simulink model "BLDC_G431"  (R2021a)
settings: Solver=FixedStepDiscrete  StartTime=0.0  StopTime=6  FixedStep=1e-6  RelTol=1e-3
values from neighbouring files (symbols this model uses):
  fpwm = 10000    [BLDC_G431_M.m]
  G1 = -4000    [BLDC_G431_M.m]
  G2 = 14000    [BLDC_G431_M.m]
  Ki = 450    [BLDC_G431_M.m]
  Kp = 0.45    [BLDC_G431_M.m]
  LBG_K1 = -4000    [BLDC_G431_M.m]
  LBG_K2 = 14000    [BLDC_G431_M.m]
  lbg_pll_w = 50    [BLDC_G431_M.m]
  lbg_speedfilter = 0.3    [BLDC_G431_M.m]
  Ld = 0.8e-3/2    (= 0.0004)    [BLDC_G431_M.m]
  Lq = 0.8e-3/2    (= 0.0004)    [BLDC_G431_M.m]
  OPL_Speed = 1200    [BLDC_G431_M.m]
  OPL_Time = 2    [BLDC_G431_M.m]
  OPL_Torque = 3    [BLDC_G431_M.m]
  Pn = 2    [BLDC_G431_M.m]
  Rs = 0.2    [BLDC_G431_M.m]
  Speed_Ki = 0.0633    [BLDC_G431_M.m]
  Speed_Kp = 0.00867    [BLDC_G431_M.m]
  Speed_PI_OutputMax = 6    [BLDC_G431_M.m]
  Speed_PI_OutputMin = -6    [BLDC_G431_M.m]
  Tpwm = 1/fpwm    (= 0.0001)    [BLDC_G431_M.m]
  UDC = 24    [BLDC_G431_M.m]
undefined symbols (not defined in the file or in its folder): Cosine_table, DiscIntNeverNeededParam, R, Sine_table, SMO_PLL_W
libraries: pid_lib x3, simulink x3, mcbplantlib x1, autolibpmsminterior x1
settings Model: DataDictionary=BLDC57.sldd  Creator=zager  LastModifiedBy=zager
settings OptimizationCC: DefaultParameterBehavior=Inlined  UseDivisionForNetSlopeComputation=on  GainParamInheritBuiltInType=on  UseFloatMulNetSlope=on  InlineInvariantSignals=on  PassReuseOutputArgsAs=Individual arguments  ZeroExternalMemoryAtStartup=off  ZeroInternalMemoryAtStartup=off  NoFixptDivByZeroProtection=on  EfficientFloat2IntCast=on  LifeSpan=1  OptimizeBlockOrder=speed  DifferentSizesBufferReuse=on  EfficientTunableParamExpr=on
settings DebuggingCC: ParameterTunabilityLossMsg=error
settings HardwareCC: ProdBitPerPointer=32  ProdBitPerSizeT=32  ProdBitPerPtrDiffT=32  ProdLargestAtomicInteger=Long  ProdLargestAtomicFloat=Double  ProdWordSize=32  ProdLongLongMode=on  ProdHWDeviceType=NXP->Cortex-M4
settings SFSimCC: MATLABDynamicMemAlloc=off
settings RTWCC: SystemTargetFile=ert.tlc  GenCodeOnly=on  TemplateMakefile=ert_default_tmf  GenerateReport=on  LaunchReport=on
settings CodeAppCC: ForceParamTrailComments=on  IgnoreCustomStorageClasses=off  OperatorAnnotations=on  SimulinkDataObjDesc=on  SFDataObjDesc=on  CustomSymbolStrGlobalVar=rt$N$M  CustomSymbolStrType=$N$M  CustomSymbolStrFcn=$N$M$F  CustomSymbolStrMacro=$N$M  InsertBlockDesc=on
settings ERTTargetCC: TargetLangStandard=C99 (ISO)  IncludeMdlTerminateFcn=off  CombineSignalStateStructs=on  SupportComplex=off  SupportNonInlinedSFcns=on  InlinedParameterPlacement=NonHierarchical  ERTCustomFileTemplate=example_file_process.tlc  ERTFilePackagingFormat=CompactWithDataFile

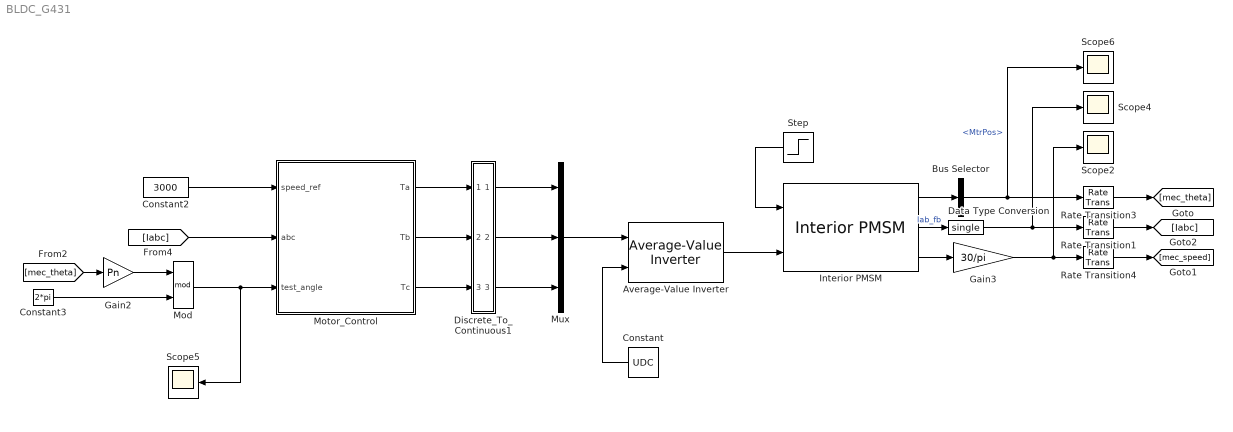
== system BLDC_G431 ==
  Average-Value Inverter : mcbplantlib/Average-Value Inverter
  Bus Selector : BusSelector  OutputSignals=MtrPos
  Constant : Constant  Value=UDC
  Constant2 : Constant  Value=3000  OutDataTypeStr=single
  Constant3 : Constant  Value=2*pi  OutDataTypeStr=single
  Data Type Conversion : DataTypeConversion  OutDataTypeStr=single
  Discrete_To_Continuous1 : Subsystem  Description=""
      mask Display: fprintf('D/C')
  Gain2 : Gain  Gain=Pn  OutDataTypeStr=single
  Gain3 : Gain  Gain=30/pi
  Interior PMSM : autolibpmsminterior/Interior PMSM  port_config=Torque  sim_type=Discrete  Ts=1e-6  P=2  Rs=0.2  Ldq=[0.4e-3 0.4e-3]  KConstText=Back-emf constant (Ke):  lambda_pm=Fluxs  Ke=6.6*sqrt(2)  mechanical=[0.5e-4,8e-5,0]  idq0=[0 0]  theta_init=0  omega_init=0  KConst=6.6*sqrt(2)  lambda_pm_calc=0.02573  Kt=0.07  RefBlkName='autolibpmsminterior/Interior PMSM'  aMode=5
      settings: SourceProductBaseCode=PW,DR,MT,UV,VE
  Mod : Math  Operator=mod  SaturateOnIntegerOverflow=on
  Motor_Control : Subsystem
  Mux : Mux  Inputs=3
  Rate Transition1 : RateTransition  OutPortSampleTime=Tpwm
  Rate Transition3 : RateTransition  OutPortSampleTime=Tpwm
  Rate Transition4 : RateTransition  OutPortSampleTime=Tpwm
  Scope{2,4..6} (4 alike) : Scope
  Step : Step  Time=3  Before=0.1  After=0  SampleTime=0
  wires:
  Constant/1 -> Average-Value Inverter/2
  Average-Value Inverter/1 -> Interior PMSM/2
  Mux/1 -> Average-Value Inverter/1
  Interior PMSM/1 -> Bus Selector/1
  Bus Selector/1 -> Rate Transition3/1, Scope6/1  "<MtrPos>"
  Data Type Conversion/1 -> Rate Transition1/1, Scope4/1
  Interior PMSM/2 -> Data Type Conversion/1  "Iab_fb"
  Discrete_To_Continuous1/1(T1) -> Mux/1
  Discrete_To_Continuous1/2(T2) -> Mux/2
  Discrete_To_Continuous1/3(T3) -> Mux/3
  Rate Transition1/1 -> [Iabc]
  Rate Transition3/1 -> [mec_theta]
  Step/1 -> Interior PMSM/1
  Constant2/1 -> Motor_Control/1(speed_ref)
  [Iabc] -> Motor_Control/2(abc)
  Motor_Control/1(Ta) -> Discrete_To_Continuous1/1(Ta)
  Motor_Control/2(Tb) -> Discrete_To_Continuous1/2(Tb)
  Motor_Control/3(Tc) -> Discrete_To_Continuous1/3(Tc)
  [mec_theta] -> Gain2/1
  Gain2/1 -> Mod/1
  Mod/1 -> Scope5/1, Motor_Control/3(test_angle)
  Rate Transition4/1 -> [mec_speed]
  Interior PMSM/3 -> Gain3/1
  Gain3/1 -> Rate Transition4/1, Scope2/1
  Constant3/1 -> Mod/2

== system BLDC_G431/Discrete_To_Continuous1 ==
  note: Discrete To Continuous
  Ta : Inport
  Tb : Inport  Port=2
  Tc : Inport  Port=3
  DT : DataTypeConversion
  DT1 : DataTypeConversion
  DT2 : DataTypeConversion
  RT : RateTransition  Integrity=off
  RT1 : RateTransition  Integrity=off
  RT2 : RateTransition  Integrity=off
  T1 : Outport
  T2 : Outport  Port=2
  T3 : Outport  Port=3
  wires:
  DT/1 -> RT/1
  Ta/1 -> DT/1  "Tabc"
  DT1/1 -> RT1/1
  Tb/1 -> DT1/1  "Tabc"
  DT2/1 -> RT2/1
  Tc/1 -> DT2/1  "Tabc"
  RT/1 -> T1/1  "Tabc"
  RT1/1 -> T2/1  "Tabc"
  RT2/1 -> T3/1  "Tabc"

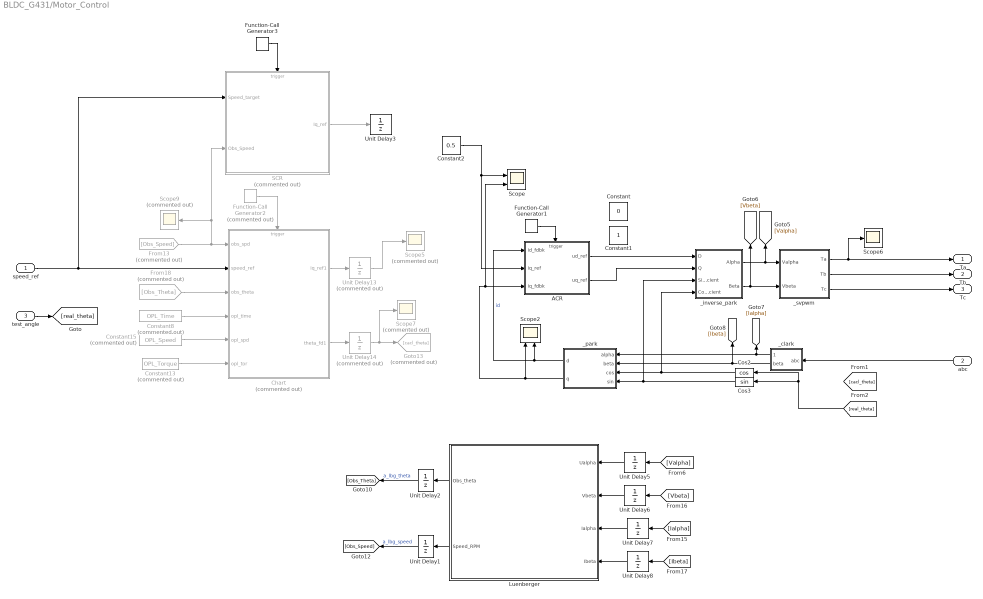
== system BLDC_G431/Motor_Control ==
  speed_ref : Inport
  abc : Inport  Port=2
  test_angle : Inport  Port=3
  ACR : Subsystem
  Chart : Stateflow chart  Commented=on  TreatAsAtomicUnit=on
  Constant : Constant  Value=0  OutDataTypeStr=single
  Constant1 : Constant  OutDataTypeStr=single
  Constant13 : Constant  Commented=on  Value=OPL_Torque  OutDataTypeStr=single
  Constant15 : Constant  Commented=on  Value=OPL_Speed  OutDataTypeStr=single
  Constant2 : Constant  Value=0.5  OutDataTypeStr=single
  Constant8 : Constant  Commented=on  Value=OPL_Time  OutDataTypeStr=single
  Cos2 : Trigonometry  Operator=cos
  Cos3 : Trigonometry
  From13 : From  Commented=on  GotoTag=Obs_Speed
  From18 : From  Commented=on  GotoTag=Obs_Theta
  Function-Call Generator1 : simulink/Ports & Subsystems/Function-Call Generator  sample_time=0.0001  numberOfIterations=1  DisallowWideOutput=off
  Function-Call Generator2 : simulink/Ports & Subsystems/Function-Call Generator  Commented=on  sample_time=0.0001  numberOfIterations=1  DisallowWideOutput=off
  Function-Call Generator3 : simulink/Ports & Subsystems/Function-Call Generator  sample_time=0.002  numberOfIterations=1  DisallowWideOutput=off
  Goto13 : Goto  Commented=on  GotoTag=cacl_theta
  Luenberger : Subsystem  TreatAsAtomicUnit=on
      settings: RTWSystemCode=Nonreusable function
  SCR : Subsystem  Commented=on  TreatAsAtomicUnit=on
      settings: FunctionInterfaceSpec=Allow arguments (Optimized)
  Scope : Scope  NumInputPorts=2
  Scope2 : Scope  NumInputPorts=2
  Scope5 : Scope  Commented=on
  Scope6 : Scope
  Scope7 : Scope  Commented=on
  Scope9 : Scope  Commented=on
  Unit Delay{1..3,5..8} (7 alike) : UnitDelay  SampleTime=-1  HasFrameUpgradeWarning=on
  Unit Delay13 : UnitDelay  Commented=on  SampleTime=-1  HasFrameUpgradeWarning=on
  Unit Delay14 : UnitDelay  Commented=on  SampleTime=-1  HasFrameUpgradeWarning=on
  _clark : Subsystem
  _inverse_park : Subsystem  TreatAsAtomicUnit=on
      settings: RTWSystemCode=Nonreusable function  RTWFcnNameOpts=Use subsystem name
      mask Display:
      | port_label('input',1,'D')
      | port_label('input',2,'Q')
      | port_label('input',3,'Sin')
      | port_label('input',4,'Cos')
      | port_label('output',1,'\alpha','texmode', 'on')
      | port_label('output',2,'\beta','texmode', 'on')
  _park : Subsystem
  _svpwm : Subsystem
  Ta : Outport
  Tb : Outport  Port=2
  Tc : Outport  Port=3
  wires:
  Cos2/1 -> _inverse_park/4(Cos_Coefficient), _park/3(cos)
  _clark/1(alpha) -> _park/1(alpha), [Ialpha]
  Chart/1(iq_ref1) -> Unit Delay13/1
  _clark/2(beta) -> _park/2(beta), [Ibeta]
  Unit Delay14/1 -> Scope7/1, Goto13/1
  Cos3/1 -> _inverse_park/3(Sin_Coefficient), _park/4(sin)
  Unit Delay6/1 -> Luenberger/2(Vbeta)
  _park/1(d) -> Scope2/2, ACR/1(id_fdbk)  "id"
  From13/1 -> Scope9/1, SCR/2(Obs_Speed), Chart/1(obs_spd)
  Chart/2(theta_fd1) -> Unit Delay14/1
  Unit Delay13/1 -> Scope5/1
  _park/2(q) -> Scope2/1, Scope/2, ACR/3(iq_fdbk)
  _inverse_park/1(Alpha) -> _svpwm/1(Valpha), [Valpha]
  [Ibeta] -> Unit Delay8/1
  [Ialpha] -> Unit Delay7/1
  _svpwm/1(Ta) -> Ta/1, Scope6/1
  Unit Delay2/1 -> [Obs_Theta]  "a_lbg_theta"
  Unit Delay7/1 -> Luenberger/3(Ialpha)
  Luenberger/2(Speed_RPM) -> Unit Delay1/1
  _inverse_park/2(Beta) -> [Vbeta], _svpwm/2(Vbeta)
  From18/1 -> Chart/3(obs_theta)
  Unit Delay8/1 -> Luenberger/4(Ibeta)
  [Vbeta] -> Unit Delay6/1
  Function-Call Generator1/1 -> ACR/Trigger
  Unit Delay5/1 -> Luenberger/1(Ualpha)
  Constant13/1 -> Chart/6(opl_tor)
  Luenberger/1(Obs_theta) -> Unit Delay2/1
  Function-Call Generator2/1 -> Chart/Trigger
  Constant8/1 -> Chart/4(opl_time)
  Unit Delay1/1 -> [Obs_Speed]  "a_lbg_speed"
  Constant15/1 -> Chart/5(opl_spd)
  [Valpha] -> Unit Delay5/1
  _svpwm/2(Tb) -> Tb/1
  _svpwm/3(Tc) -> Tc/1
  abc/1 -> _clark/1(abc)
  speed_ref/1 -> Chart/2(speed_ref), SCR/1(Speed_target)
  test_angle/1 -> [real_theta]
  ACR/1(ud_ref) -> _inverse_park/1(D)
  ACR/2(uq_ref) -> _inverse_park/2(Q)
  Function-Call Generator3/1 -> SCR/Trigger
  SCR/1(Iq_ref) -> Unit Delay3/1
  Constant2/1 -> ACR/2(iq_ref), Scope/1
  [real_theta] -> Cos3/1, Cos2/1

== system BLDC_G431/Motor_Control/ACR ==
  id_fdbk : Inport
  iq_ref : Inport  Port=2
  iq_fdbk : Inport  Port=3
  function : TriggerPort  TriggerType=function-call  VariantControl=(inherit)  SampleTimeType=periodic  SampleTime=-1
  Constant : Constant  Value=0  OutDataTypeStr=single
  PID Controller1 : pid_lib/PID Controller  Controller=PI  Form=Parallel  TimeDomain=Discrete-time  UseExternalTs=off  SampleTime=-1  IntegratorMethod=Forward Euler  FilterMethod=Forward Euler  ControllerParametersSource=internal  P=Kp  I=Ki  D=0  UseFilter=on  N=100  TunerSelectOption=Transfer Function Based (PID Tuner App)  InitialConditionSource=internal  InitialConditionForIntegrator=0  InitialConditionForFilter=0  DifferentiatorICPrevScaledInput=0  ExternalReset=none  TrackingMode=off  Kt=1  LimitOutput=on  SatLimitsSource=internal  UpperSaturationLimit=24*0.9/sqrt(3)  LowerSaturationLimit=-24*0.9/sqrt(3)  LinearizeAsGain=on  AntiWindupMode=clamping  Kb=1  PGainOutDataTypeStr=single  PProdOutDataTypeStr=single  POutMin=[]  POutMax=[]  IGainOutDataTypeStr=single  IProdOutDataTypeStr=single  IOutMin=[]  IOutMax=[]  DOutMin=[]  DOutMax=[]  NOutMin=[]  NOutMax=[]  SumOutDataTypeStr=single  SumOutMin=[]  SumOutMax=[]  SaturationOutDataTypeStr=single  SaturationOutMin=[]  SaturationOutMax=[]  PParamMin=[]  PParamMax=[]  IParamMin=[]  IParamMax=[]  DParamMin=[]  DParamMax=[]  NParamMin=[]  NParamMax=[]  KbParamMin=[]  KbParamMax=[]  KtParamMin=[]  KtParamMax=[]  KbOutMin=[]  KbOutMax=[]  KtOutMin=[]  KtOutMax=[]  IntegratorOutMin=[]  IntegratorOutMax=[]  FilterOutMin=[]  FilterOutMax=[]  SumI1OutMin=[]  SumI1OutMax=[]  SumI2OutMin=[]  SumI2OutMax=[]  SumI3OutMin=[]  SumI3OutMax=[]  SumI4OutMin=[]  SumI4OutMax=[]  SumDOutMin=[]  SumDOutMax=[]  DifferentiatorOutMin=[]  DifferentiatorOutMax=[]  FilterDiffOutCoefMin=[]  FilterDiffOutCoefMax=[]  ReciprocalOutMin=[]  ReciprocalOutMax=[]  SumDenOutMin=[]  SumDenOutMax=[]  SumNumOutMin=[]  SumNumOutMax=[]  DivideOutMin=[]  DivideOutMax=[]  UdiffTsProdOutMin=[]  UdiffTsProdOutMax=[]  NTsProdOutMin=[]  NTsProdOutMax=[]  UintegralTsProdOutMin=[]  UintegralTsProdOutMax=[]  UngainTsProdOutMin=[]  UngainTsProdOutMax=[]  IntegratorContinuousStateAttributes=''  IntegratorStateMustResolveToSignalObject=off  IntegratorRTWStateStorageClass=Auto  FilterContinuousStateAttributes=''  FilterStateMustResolveToSignalObject=off  FilterRTWStateStorageClass=Auto  ParallelPVariant=InternalParameters  IdealPVariant=Disabled  IVariant=InternalParameters  DVariant=Disabled  IntegratorVariant=Discrete  SatVariant=Enabled  AWVariant=DiscClampingParallel  PCopyVariant=Disabled  TRVariant=Disabled  FdbkBlocksVariant=Forward  IdealPFdbkVariant=Disabled  SatFdbkVariant=Disabled  DerivativeFilterVariant=Disabled  NVariant=Disabled  NCopyVariant=Disabled_SignalSpec  FilterICVariant=Disabled  IntegratorICVariant=InternalICs  ExternalResetVariant=Disabled  TRSumVariant=Passthrough  SumFdbkVariant=Disabled  SumVariant=Sum_PI  TsampFilterVariant=InternalTs  TsampNgainVariant=Passthrough  TsampIntegralVariant=Passthrough  ExternalSaturationOutDataTypeStr=Inherit: Same as second input
  PID Controller2 : pid_lib/PID Controller  Controller=PI  Form=Parallel  TimeDomain=Discrete-time  UseExternalTs=off  SampleTime=-1  IntegratorMethod=Forward Euler  FilterMethod=Forward Euler  ControllerParametersSource=internal  P=Kp  I=Ki  D=0  UseFilter=on  N=100  TunerSelectOption=Transfer Function Based (PID Tuner App)  InitialConditionSource=internal  InitialConditionForIntegrator=0  InitialConditionForFilter=0  DifferentiatorICPrevScaledInput=0  ExternalReset=none  TrackingMode=off  Kt=1  LimitOutput=on  SatLimitsSource=internal  UpperSaturationLimit=24*0.9/sqrt(3)  LowerSaturationLimit=-24*0.9/sqrt(3)  LinearizeAsGain=on  AntiWindupMode=clamping  Kb=1  PGainOutDataTypeStr=single  PProdOutDataTypeStr=single  POutMin=[]  POutMax=[]  IGainOutDataTypeStr=single  IProdOutDataTypeStr=single  IOutMin=[]  IOutMax=[]  DOutMin=[]  DOutMax=[]  NOutMin=[]  NOutMax=[]  SumOutDataTypeStr=single  SumOutMin=[]  SumOutMax=[]  SaturationOutDataTypeStr=single  SaturationOutMin=[]  SaturationOutMax=[]  PParamMin=[]  PParamMax=[]  IParamMin=[]  IParamMax=[]  DParamMin=[]  DParamMax=[]  NParamMin=[]  NParamMax=[]  KbParamMin=[]  KbParamMax=[]  KtParamMin=[]  KtParamMax=[]  KbOutMin=[]  KbOutMax=[]  KtOutMin=[]  KtOutMax=[]  IntegratorOutMin=[]  IntegratorOutMax=[]  FilterOutMin=[]  FilterOutMax=[]  SumI1OutMin=[]  SumI1OutMax=[]  SumI2OutMin=[]  SumI2OutMax=[]  SumI3OutMin=[]  SumI3OutMax=[]  SumI4OutMin=[]  SumI4OutMax=[]  SumDOutMin=[]  SumDOutMax=[]  DifferentiatorOutMin=[]  DifferentiatorOutMax=[]  FilterDiffOutCoefMin=[]  FilterDiffOutCoefMax=[]  ReciprocalOutMin=[]  ReciprocalOutMax=[]  SumDenOutMin=[]  SumDenOutMax=[]  SumNumOutMin=[]  SumNumOutMax=[]  DivideOutMin=[]  DivideOutMax=[]  UdiffTsProdOutMin=[]  UdiffTsProdOutMax=[]  NTsProdOutMin=[]  NTsProdOutMax=[]  UintegralTsProdOutMin=[]  UintegralTsProdOutMax=[]  UngainTsProdOutMin=[]  UngainTsProdOutMax=[]  IntegratorContinuousStateAttributes=''  IntegratorStateMustResolveToSignalObject=off  IntegratorRTWStateStorageClass=Auto  FilterContinuousStateAttributes=''  FilterStateMustResolveToSignalObject=off  FilterRTWStateStorageClass=Auto  ParallelPVariant=InternalParameters  IdealPVariant=Disabled  IVariant=InternalParameters  DVariant=Disabled  IntegratorVariant=Discrete  SatVariant=Enabled  AWVariant=DiscClampingParallel  PCopyVariant=Disabled  TRVariant=Disabled  FdbkBlocksVariant=Forward  IdealPFdbkVariant=Disabled  SatFdbkVariant=Disabled  DerivativeFilterVariant=Disabled  NVariant=Disabled  NCopyVariant=Disabled_SignalSpec  FilterICVariant=Disabled  IntegratorICVariant=InternalICs  ExternalResetVariant=Disabled  TRSumVariant=Passthrough  SumFdbkVariant=Disabled  SumVariant=Sum_PI  TsampFilterVariant=InternalTs  TsampNgainVariant=Passthrough  TsampIntegralVariant=Passthrough  ExternalSaturationOutDataTypeStr=Inherit: Same as second input
  Scope : Scope  NumInputPorts=2
  Scope1 : Scope
  Sum1 : Sum  Inputs=|+-
  Sum7 : Sum  Inputs=|+-
  ud_ref : Outport
  uq_ref : Outport  Port=2
  wires:
  Constant/1 -> Sum1/1
  Sum1/1 -> PID Controller1/1
  Sum7/1 -> Scope1/1, PID Controller2/1
  PID Controller1/1 -> Scope/1, ud_ref/1
  PID Controller2/1 -> Scope/2, uq_ref/1
  iq_ref/1 -> Sum7/1
  id_fdbk/1 -> Sum1/2
  iq_fdbk/1 -> Sum7/2

== system BLDC_G431/Motor_Control/Chart/close_loop ==
  obs_spd : Inport  OutDataTypeStr=single  PortDimensions=1
  obs_theta : Inport  Port=2  OutDataTypeStr=single  PortDimensions=1
  speed_ref : Inport  Port=3  OutDataTypeStr=single  PortDimensions=1
  f : TriggerPort  TriggerType=function-call  VariantControl=(inherit)  SampleTime=0.002
      settings: CopyFcn=Stateflow.SLINSF.SimulinkMan.removeBlockPreDeleteFcn  PreDeleteFcn=Stateflow.SLINSF.SimulinkMan.unsafePredeleteFcn
  Constant : Constant  Value=0.5  OutDataTypeStr=single
  Data Type Conversion : DataTypeConversion  OutDataTypeStr=single
  SCR : Subsystem  TreatAsAtomicUnit=on
      settings: FunctionInterfaceSpec=Allow arguments (Optimized)
  Scope : Scope
  Scope1 : Scope
  Step : Step  Time=3  Before=0.8  After=0.5
  theta_fd1 : Outport  OutDataTypeStr=single
  iq_ref1 : Outport  Port=2  OutDataTypeStr=single
  wires:
  speed_ref/1 -> SCR/1(Speed_target)
  obs_spd/1 -> SCR/2(Obs_Speed)
  obs_theta/1 -> Scope/1, theta_fd1/1
  Data Type Conversion/1 -> Scope1/1
  Step/1 -> Data Type Conversion/1
  SCR/1(Iq_ref) -> iq_ref1/1

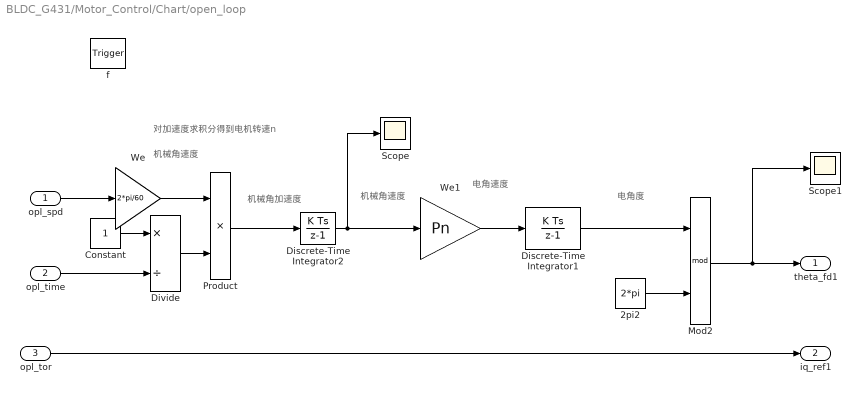
== system BLDC_G431/Motor_Control/Chart/open_loop ==
  note: 电角度
  note: 电角速度
  note: 机械角速度
  note: 机械角速度
  note: 机械角加速度
  note: 对加速度求积分得到电机转速n
  opl_spd : Inport  OutDataTypeStr=single  PortDimensions=1
  opl_time : Inport  Port=2  OutDataTypeStr=single  PortDimensions=1
  opl_tor : Inport  Port=3  OutDataTypeStr=single  PortDimensions=1
  f : TriggerPort  TriggerType=function-call  VariantControl=(inherit)
      settings: CopyFcn=Stateflow.SLINSF.SimulinkMan.removeBlockPreDeleteFcn  PreDeleteFcn=Stateflow.SLINSF.SimulinkMan.unsafePredeleteFcn
  2pi2 : Constant  Value=2*pi  OutDataTypeStr=single
  Constant : Constant  OutDataTypeStr=single
  Discrete-Time Integrator1 : DiscreteIntegrator  SampleTime=-1  ICPrevOutput=DiscIntNeverNeededParam  ICPrevScaledInput=DiscIntNeverNeededParam
  Discrete-Time Integrator2 : DiscreteIntegrator  SampleTime=-1  ICPrevOutput=DiscIntNeverNeededParam  ICPrevScaledInput=DiscIntNeverNeededParam
  Divide : Product  Inputs=*/
  Mod2 : Math  Operator=mod  SaturateOnIntegerOverflow=on
  Product : Product
  Scope : Scope
  Scope1 : Scope
  We : Gain  Gain=2*pi/60  OutDataTypeStr=single  ParamDataTypeStr=Inherit: Same as input
  We1 : Gain  Gain=Pn  OutDataTypeStr=single  ParamDataTypeStr=Inherit: Same as input
  theta_fd1 : Outport  OutDataTypeStr=single
  iq_ref1 : Outport  Port=2  OutDataTypeStr=single
  wires:
  Constant/1 -> Divide/1
  Divide/1 -> Product/2
  2pi2/1 -> Mod2/2
  opl_time/1 -> Divide/2
  Product/1 -> Discrete-Time Integrator2/1
  Mod2/1 -> Scope1/1, theta_fd1/1
  opl_spd/1 -> We/1
  Discrete-Time Integrator1/1 -> Mod2/1
  Discrete-Time Integrator2/1 -> We1/1, Scope/1
  opl_tor/1 -> iq_ref1/1
  We1/1 -> Discrete-Time Integrator1/1
  We/1 -> Product/1

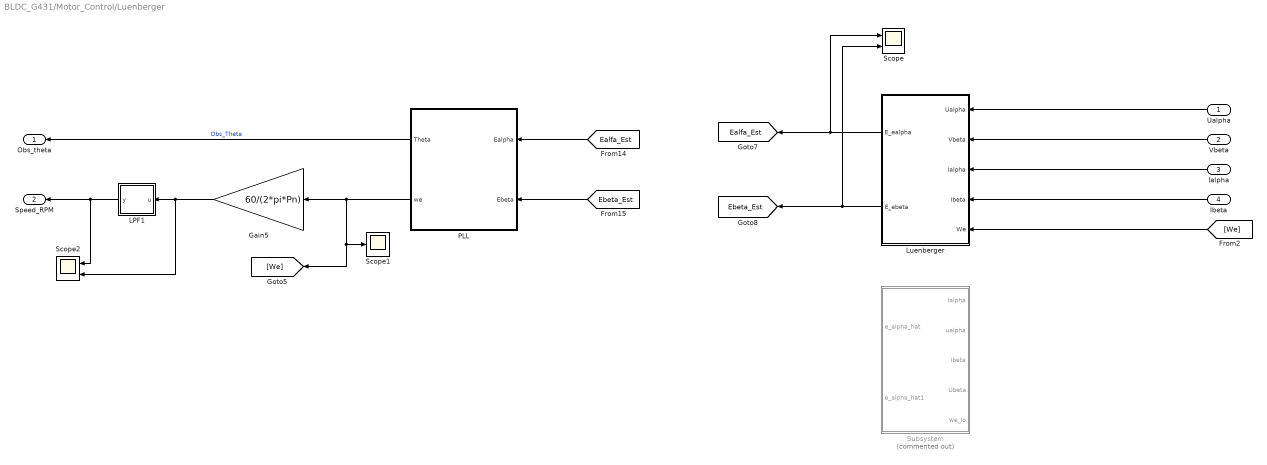
== system BLDC_G431/Motor_Control/Luenberger ==
  Ualpha : Inport
  Vbeta : Inport  Port=2
  Ialpha : Inport  Port=3
  Ibeta : Inport  Port=4
  Gain5 : Gain  Gain=60/(2*pi*Pn)
  LPF1 : Subsystem
  Luenberger : Subsystem
  PLL : Subsystem
  Scope : Scope  NumInputPorts=2
  Scope1 : Scope
  Scope2 : Scope  NumInputPorts=2
  Subsystem : Subsystem  Commented=on
  Obs_theta : Outport
  Speed_RPM : Outport  Port=2
  tag scope: Ealfa_Est=global, Ebeta_Est=global
  wires:
  Ibeta/1 -> Luenberger/4(Ibeta)
  Vbeta/1 -> Luenberger/2(Vbeta)
  Ialpha/1 -> Luenberger/3(Ialpha)
  Ualpha/1 -> Luenberger/1(Ualpha)
  [Ebeta_Est] -> PLL/2(Ebeta)
  [Ealfa_Est] -> PLL/1(Ealpha)
  Gain5/1 -> Scope2/2, LPF1/1(u)
  PLL/1(Theta) -> Obs_theta/1  "Obs_Theta"
  LPF1/1(y) -> Scope2/1, Speed_RPM/1
  Luenberger/1(E_ealpha) -> Scope/1, [Ealfa_Est]
  Luenberger/2(E_ebeta) -> Scope/2, [Ebeta_Est]
  [We] -> Luenberger/5(We)
  PLL/2(we) -> Scope1/1, [We], Gain5/1

== system BLDC_G431/Motor_Control/SCR ==
  Speed_target : Inport
  Obs_Speed : Inport  Port=2  OutMin=0  OutMax=2*pi  OutDataTypeStr=single
  function : TriggerPort  TriggerType=function-call  VariantControl=(inherit)  SampleTimeType=periodic  SampleTime=-1
  Constant1 : Constant  Value=0  OutDataTypeStr=uint8
  PI : Subsystem
  Scope : Scope  NumInputPorts=2
  Scope1 : Scope
  Sum : Sum  Inputs=|+-
  Iq_ref : Outport  OutDataTypeStr=single
  wires:
  Obs_Speed/1 -> Scope/2, Sum/2
  Speed_target/1 -> Scope/1, Sum/1
  Constant1/1 -> PI/2(Reset)
  Sum/1 -> PI/1(Err)
  PI/1(PI_Out) -> Scope1/1, Iq_ref/1

== system BLDC_G431/Motor_Control/_clark ==
  abc : Inport
  Add : Sum  Inputs=+--
  Add1 : Sum  Inputs=+-
  Demux : Demux  Outputs=3
  Gain : Gain  Gain=0.5
  Gain1 : Gain  Gain=0.5
  Gain2 : Gain  Gain=2/3
  Gain3 : Gain  Gain=sqrt(3)/2
  Gain4 : Gain  Gain=sqrt(3)/2
  Gain5 : Gain  Gain=2/3
  alpha : Outport
  beta : Outport  Port=2
  wires:
  Demux/1 -> Add/1
  Demux/3 -> Gain4/1, Gain1/1
  Gain3/1 -> Add1/1
  abc/1 -> Demux/1
  Gain1/1 -> Add/3
  Add/1 -> Gain2/1
  Gain5/1 -> beta/1
  Demux/2 -> Gain3/1, Gain/1
  Add1/1 -> Gain5/1
  Gain2/1 -> alpha/1
  Gain/1 -> Add/2
  Gain4/1 -> Add1/2

== system BLDC_G431/Motor_Control/_inverse_park ==
  D : Inport
  Q : Inport  Port=2
  Sin_Coefficient : Inport  Port=3
  Cos_Coefficient : Inport  Port=4
  Add1 : Sum  Inputs=+-  OutDataTypeStr=Inherit: Same as first input
  Add2 : Sum  OutDataTypeStr=Inherit: Same as first input
  Cos_Coefficient1 : InportShadow  Port=4
  Product{1..4} (4 alike) : Product  RndMeth=Simplest  OutDataTypeStr=Inherit: Same as first input
  Sin_Coefficient1 : InportShadow  Port=3
  Alpha : Outport  VectorParamsAs1DForOutWhenUnconnected=off
  Beta : Outport  Port=2  VectorParamsAs1DForOutWhenUnconnected=off
  wires:
  Product3/1 -> Add2/1
  Product4/1 -> Add2/2
  Product1/1 -> Add1/1
  Product2/1 -> Add1/2
  Cos_Coefficient1/1 -> Product4/2
  Sin_Coefficient/1 -> Product2/2
  D/1 -> Product3/1, Product1/1
  Q/1 -> Product2/1, Product4/1
  Sin_Coefficient1/1 -> Product3/2
  Cos_Coefficient/1 -> Product1/2
  Add1/1 -> Alpha/1
  Add2/1 -> Beta/1

== system BLDC_G431/Motor_Control/_park ==
  alpha : Inport
  beta : Inport  Port=2
  cos : Inport  Port=3
  sin : Inport  Port=4
  Add1 : Sum  OutDataTypeStr=Inherit: Same as first input
  Add2 : Sum  Inputs=-+  OutDataTypeStr=Inherit: Same as first input
  Produc3t : Product  RndMeth=Simplest  OutDataTypeStr=Inherit: Same as first input
  Product1 : Product  RndMeth=Simplest  OutDataTypeStr=Inherit: Same as first input
  Product2 : Product  RndMeth=Simplest  OutDataTypeStr=Inherit: Same as first input
  Product4 : Product  RndMeth=Simplest  OutDataTypeStr=Inherit: Same as first input
  d : Outport
  q : Outport  Port=2
  wires:
  alpha/1 -> Product1/1, Produc3t/1
  Add1/1 -> d/1
  Product2/1 -> Add1/2
  beta/1 -> Product2/1, Product4/2
  Add2/1 -> q/1
  Product4/1 -> Add2/2
  sin/1 -> Product2/2, Produc3t/2
  cos/1 -> Product1/2, Product4/1
  Produc3t/1 -> Add2/1
  Product1/1 -> Add1/1

== system BLDC_G431/Motor_Control/_svpwm ==
  Valpha : Inport
  Vbeta : Inport  Port=2
  Constant : Constant  Value=UDC
  Constant4 : Constant  Value=Tpwm  OutDataTypeStr=single
  N Sector  Caculate : Subsystem  TreatAsAtomicUnit=on
  Subsystem : Subsystem
  Subsystem1 : Subsystem
  Subsystem2 : Subsystem
  T1 T2  Caculate : Subsystem  TreatAsAtomicUnit=on
  Tcm calculate : Subsystem  TreatAsAtomicUnit=on
  XYZ Caculate : Subsystem  TreatAsAtomicUnit=on
  Ta : Outport
  Tb : Outport  Port=2
  Tc : Outport  Port=3
  wires:
  Tcm calculate/2(Tcm2) -> Subsystem1/1(Tb)
  Subsystem2/1(Dc) -> Tc/1
  Subsystem/1(Da) -> Ta/1
  Tcm calculate/1(Tcm1) -> Subsystem/1(Ta)
  XYZ Caculate/3(Z) -> T1 T2  Caculate/4(Z)
  Subsystem1/1(Db) -> Tb/1
  Valpha/1 -> N Sector  Caculate/2(Ualf), XYZ Caculate/1(Ualfpa)
  Constant4/1 -> XYZ Caculate/4(Tpwm), Tcm calculate/4(Tpwm), T1 T2  Caculate/5(Tpwm)
  XYZ Caculate/2(Y) -> T1 T2  Caculate/3(Y)
  XYZ Caculate/1(X) -> T1 T2  Caculate/2(X)
  N Sector  Caculate/1(N) -> T1 T2  Caculate/1(N), Tcm calculate/1(N)
  Vbeta/1 -> N Sector  Caculate/1(Ubelta), XYZ Caculate/2(Ubelta)
  T1 T2  Caculate/2(T2) -> Tcm calculate/3(T2)
  T1 T2  Caculate/1(T1) -> Tcm calculate/2(T1)
  Tcm calculate/3(Tcm3) -> Subsystem2/1(Tc)
  Constant/1 -> XYZ Caculate/3(Udc)

== system BLDC_G431/Motor_Control/Chart/close_loop/SCR ==
  Speed_target : Inport
  Obs_Speed : Inport  Port=2  OutMin=0  OutMax=2*pi  OutDataTypeStr=single
  Constant1 : Constant  Value=0  OutDataTypeStr=uint8
  PI : Subsystem
  Scope : Scope  NumInputPorts=2
  Scope1 : Scope
  Sum : Sum  Inputs=|+-
  Iq_ref : Outport  OutDataTypeStr=single
  wires:
  Obs_Speed/1 -> Scope/2, Sum/2
  Speed_target/1 -> Scope/1, Sum/1
  Constant1/1 -> PI/2(Reset)
  Sum/1 -> PI/1(Err)
  PI/1(PI_Out) -> Scope1/1, Iq_ref/1

== system BLDC_G431/Motor_Control/Luenberger/LPF1 ==
  u : Inport
  Add : Sum  Inputs=+-
  Add1 : Sum
  Constant1 : Constant  Value=lbg_speedfilter  OutDataTypeStr=single
  Divide1 : Product  Inputs=**
  Unit Delay : UnitDelay  SampleTime=-1  HasFrameUpgradeWarning=on
  y : Outport
  wires:
  Constant1/1 -> Divide1/1
  u/1 -> Add/1
  Add/1 -> Divide1/2
  Divide1/1 -> Add1/1
  Unit Delay/1 -> Add/2, Add1/2
  Add1/1 -> Unit Delay/1, y/1

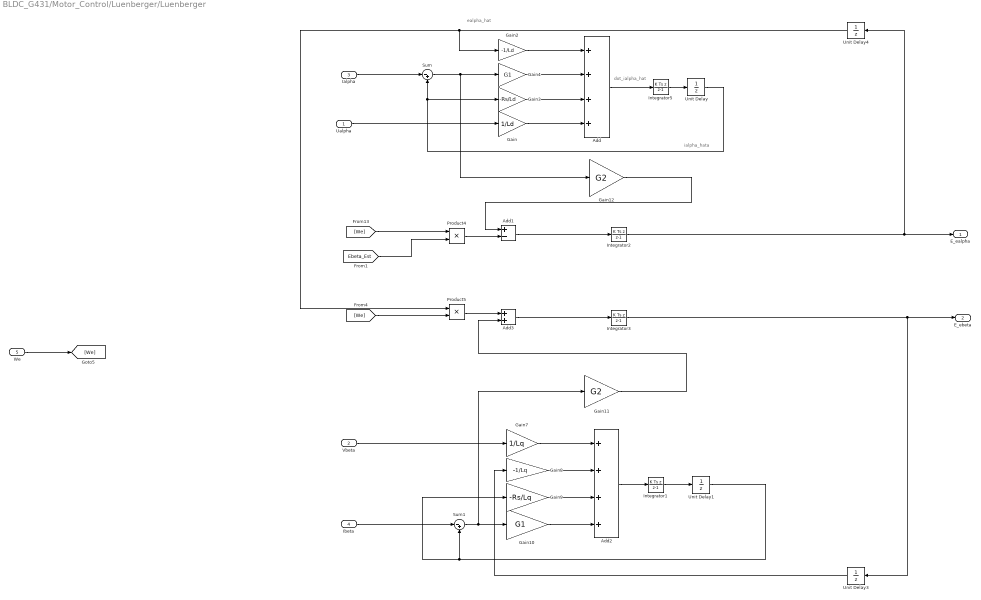
== system BLDC_G431/Motor_Control/Luenberger/Luenberger ==
  note: dot_ialpha_hat
  note: ialpha_hata
  note: ealpha_hat
  Ualpha : Inport
  Vbeta : Inport  Port=2
  Ialpha : Inport  Port=3
  Ibeta : Inport  Port=4
  We : Inport  Port=5
  Add : Sum  Inputs=++++
  Add1 : Sum  Inputs=+-
  Add2 : Sum  Inputs=++++
  Add3 : Sum
  Gain : Gain  Gain=1/Ld
  Gain10 : Gain  Gain=G1
  Gain11 : Gain  Gain=G2
  Gain12 : Gain  Gain=G2
  Gain2 : Gain  Gain=-1/Ld
  Gain3 : Gain  Gain=-Rs/Ld
  Gain4 : Gain  Gain=G1
  Gain7 : Gain  Gain=1/Lq
  Gain8 : Gain  Gain=-1/Lq
  Gain9 : Gain  Gain=-Rs/Lq
  Integrator1 : DiscreteIntegrator  IntegratorMethod=Integration: Backward Euler  SampleTime=-1  ICPrevOutput=DiscIntNeverNeededParam  ICPrevScaledInput=DiscIntNeverNeededParam  mask(DiscretizedDiscreteIntegrator){}
      mask init:
      | %tustin
  Integrator2 : DiscreteIntegrator  IntegratorMethod=Integration: Backward Euler  SampleTime=-1  ICPrevOutput=DiscIntNeverNeededParam  ICPrevScaledInput=DiscIntNeverNeededParam  mask(DiscretizedDiscreteIntegrator){}
      mask init:
      | %tustin
  Integrator3 : DiscreteIntegrator  IntegratorMethod=Integration: Backward Euler  SampleTime=-1  ICPrevOutput=DiscIntNeverNeededParam  ICPrevScaledInput=DiscIntNeverNeededParam  mask(DiscretizedDiscreteIntegrator){}
      mask init:
      | %tustin
  Integrator5 : DiscreteIntegrator  IntegratorMethod=Integration: Backward Euler  SampleTime=-1  ICPrevOutput=DiscIntNeverNeededParam  ICPrevScaledInput=DiscIntNeverNeededParam  mask(DiscretizedDiscreteIntegrator){}
      mask init:
      | %tustin
  Product4 : Product
  Product5 : Product
  Sum : Sum  Inputs=|-+
  Sum1 : Sum  Inputs=|-+
  Unit Delay{,1,3..4} (4 alike) : UnitDelay  SampleTime=-1  HasFrameUpgradeWarning=on
  E_ealpha : Outport
  E_ebeta : Outport  Port=2
  wires:
  Add2/1 -> Integrator1/1
  Integrator1/1 -> Unit Delay1/1
  Vbeta/1 -> Gain7/1
  Integrator3/1 -> E_ebeta/1, Unit Delay3/1
  Add1/1 -> Integrator2/1
  Integrator2/1 -> E_ealpha/1, Unit Delay4/1
  Gain11/1 -> Add3/2
  Product5/1 -> Add3/1
  [Ebeta_Est] -> Product4/2
  Gain10/1 -> Add2/4
  Gain8/1 -> Add2/2
  Gain9/1 -> Add2/3
  Sum1/1 -> Gain10/1, Gain11/1
  [We] -> Product5/2
  [We] -> Product4/1
  Gain7/1 -> Add2/1
  Sum/1 -> Gain4/1, Gain12/1
  Ialpha/1 -> Sum/1
  Integrator5/1 -> Unit Delay/1
  Ibeta/1 -> Sum1/1
  Add/1 -> Integrator5/1
  Ualpha/1 -> Gain/1
  Add3/1 -> Integrator3/1
  We/1 -> [We]
  Unit Delay1/1 -> Sum1/2, Gain9/1
  Unit Delay/1 -> Sum/2, Gain3/1
  Unit Delay4/1 -> Gain2/1, Product5/1
  Unit Delay3/1 -> Gain8/1
  Gain2/1 -> Add/1
  Gain3/1 -> Add/3
  Gain4/1 -> Add/2
  Gain/1 -> Add/4
  Product4/1 -> Add1/2
  Gain12/1 -> Add1/1

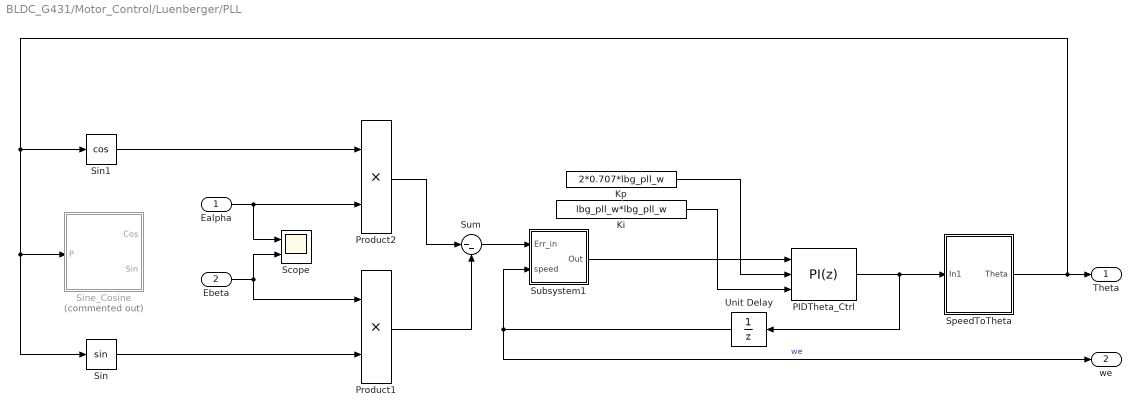
== system BLDC_G431/Motor_Control/Luenberger/PLL ==
  Ealpha : Inport
  Ebeta : Inport  Port=2
  Ki : Constant  Value=lbg_pll_w*lbg_pll_w  OutDataTypeStr=single
  Kp : Constant  Value=2*0.707*lbg_pll_w  OutDataTypeStr=single
  PIDTheta_Ctrl : pid_lib/PID Controller  Controller=PI  Form=Parallel  TimeDomain=Discrete-time  UseExternalTs=off  SampleTime=-1  IntegratorMethod=Forward Euler  FilterMethod=Forward Euler  ControllerParametersSource=external  P=2*0.707*SMO_PLL_W  I=SMO_PLL_W*SMO_PLL_W  D=0  UseFilter=on  N=100  TunerSelectOption=Transfer Function Based (PID Tuner App)  ZeroCross=off  InitialConditionSource=internal  InitialConditionForIntegrator=1  InitialConditionForFilter=0  DifferentiatorICPrevScaledInput=0  ExternalReset=none  TrackingMode=off  Kt=1  LimitOutput=on  SatLimitsSource=internal  UpperSaturationLimit=2*pi*500  LowerSaturationLimit=-2*pi*500  LinearizeAsGain=off  AntiWindupMode=clamping  Kb=50  POutMin=[]  POutMax=[]  IOutMin=[]  IOutMax=[]  DOutMin=[]  DOutMax=[]  NOutMin=[]  NOutMax=[]  SumOutMin=[]  SumOutMax=[]  SaturationOutDataTypeStr=Inherit: Inherit via back propagation  SaturationOutMin=[]  SaturationOutMax=[]  PParamMin=[]  PParamMax=[]  IParamMin=[]  IParamMax=[]  DParamMin=[]  DParamMax=[]  NParamMin=[]  NParamMax=[]  KbParamMin=[]  KbParamMax=[]  KtParamMin=[]  KtParamMax=[]  KbOutMin=[]  KbOutMax=[]  KtOutMin=[]  KtOutMax=[]  IntegratorOutMin=[]  IntegratorOutMax=[]  FilterOutMin=[]  FilterOutMax=[]  SumI1OutMin=[]  SumI1OutMax=[]  SumI2OutMin=[]  SumI2OutMax=[]  SumI3OutMin=[]  SumI3OutMax=[]  SumI4OutMin=[]  SumI4OutMax=[]  SumDOutMin=[]  SumDOutMax=[]  DifferentiatorOutMin=[]  DifferentiatorOutMax=[]  FilterDiffOutCoefMin=[]  FilterDiffOutCoefMax=[]  ReciprocalOutMin=[]  ReciprocalOutMax=[]  SumDenOutMin=[]  SumDenOutMax=[]  SumNumOutMin=[]  SumNumOutMax=[]  DivideOutMin=[]  DivideOutMax=[]  UdiffTsProdOutMin=[]  UdiffTsProdOutMax=[]  NTsProdOutMin=[]  NTsProdOutMax=[]  UintegralTsProdOutMin=[]  UintegralTsProdOutMax=[]  UngainTsProdOutMin=[]  UngainTsProdOutMax=[]  IntegratorContinuousStateAttributes=''  IntegratorStateMustResolveToSignalObject=off  IntegratorRTWStateStorageClass=Auto  FilterContinuousStateAttributes=''  FilterStateMustResolveToSignalObject=off  FilterRTWStateStorageClass=Auto  ParallelPVariant=ExternalParameters  IdealPVariant=Disabled  IVariant=ExternalParameters  DVariant=Disabled  IntegratorVariant=Discrete  SatVariant=Enabled  AWVariant=DiscClampingParallel  PCopyVariant=Disabled  TRVariant=Disabled  FdbkBlocksVariant=Forward  IdealPFdbkVariant=Disabled  SatFdbkVariant=Disabled  DerivativeFilterVariant=Disabled  NVariant=Disabled  NCopyVariant=Disabled_SignalSpec  FilterICVariant=Disabled  IntegratorICVariant=InternalICs  ExternalResetVariant=Disabled  TRSumVariant=Passthrough  SumFdbkVariant=Disabled  SumVariant=Sum_PI  TsampFilterVariant=InternalTs  TsampNgainVariant=Passthrough  TsampIntegralVariant=Passthrough  ExternalSaturationOutDataTypeStr=Inherit: Same as second input
  Product1 : Product
  Product2 : Product
  Scope : Scope  NumInputPorts=2
  Sin : Trigonometry
  Sin1 : Trigonometry  Operator=cos
  Sine_Cosine : Subsystem  Commented=on  TreatAsAtomicUnit=on
      settings: RTWSystemCode=Nonreusable function  RTWFcnNameOpts=Use subsystem name
  SpeedToTheta : Subsystem
  Subsystem1 : Subsystem
  Sum : Sum  Inputs=|--
  Unit Delay : UnitDelay  SampleTime=-1  HasFrameUpgradeWarning=on
  Theta : Outport
  we : Outport  Port=2
  wires:
  Subsystem1/1(Out) -> PIDTheta_Ctrl/1
  Sum/1 -> Subsystem1/1(Err_in)
  Product1/1 -> Sum/2
  Product2/1 -> Sum/1
  Ebeta/1 -> Scope/2, Product1/1
  Ealpha/1 -> Scope/1, Product2/2
  Unit Delay/1 -> we/1, Subsystem1/2(speed)  "we"
  PIDTheta_Ctrl/1 -> SpeedToTheta/1(In1), Unit Delay/1
  Kp/1 -> PIDTheta_Ctrl/2
  Ki/1 -> PIDTheta_Ctrl/3
  SpeedToTheta/1(Theta) -> Sin/1, Sine_Cosine/1(P), Sin1/1, Theta/1
  Sin1/1 -> Product2/1
  Sin/1 -> Product1/2

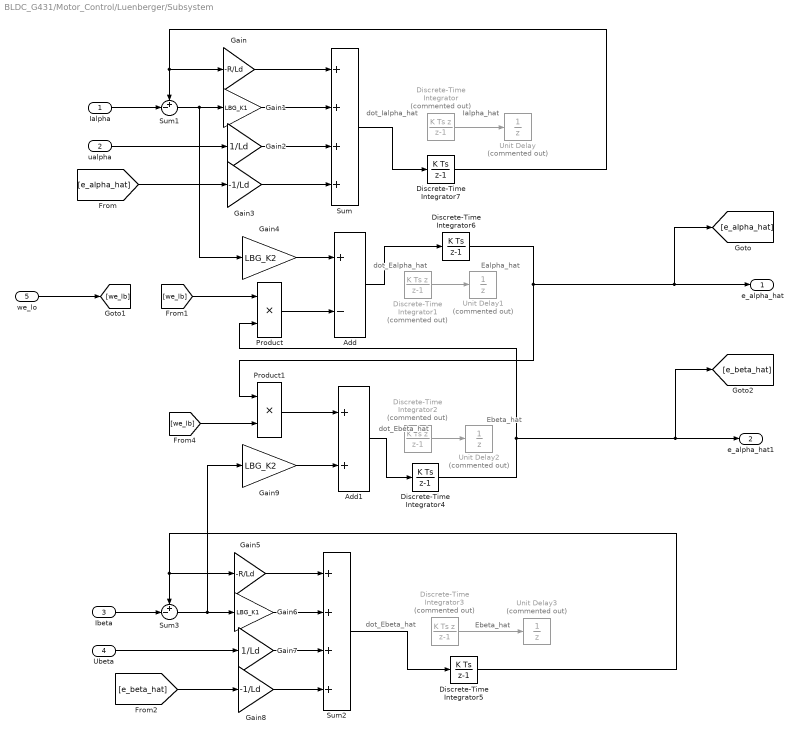
== system BLDC_G431/Motor_Control/Luenberger/Subsystem ==
  note: dot_Ealpha_hat
  note: Ialpha_hat
  note: dot_Ialpha_hat
  note: Ealpha_hat
  note: Ebeta_hat
  note: dot_Ebeta_hat
  note: dot_Ebeta_hat
  note: Ebeta_hat
  Ialpha : Inport
  ualpha : Inport  Port=2
  Ibeta : Inport  Port=3
  Ubeta : Inport  Port=4
  we_lo : Inport  Port=5
  Add : Sum  Inputs=+-
  Add1 : Sum
  Discrete-Time Integrator{,1..3} (4 alike) : DiscreteIntegrator  Commented=on  IntegratorMethod=Integration: Backward Euler  SampleTime=-1  ICPrevOutput=DiscIntNeverNeededParam  ICPrevScaledInput=DiscIntNeverNeededParam
  Discrete-Time Integrator{4..7} (4 alike) : DiscreteIntegrator  SampleTime=-1  ICPrevOutput=DiscIntNeverNeededParam  ICPrevScaledInput=DiscIntNeverNeededParam
  Gain : Gain  Gain=-R/Ld
  Gain1 : Gain  Gain=LBG_K1
  Gain2 : Gain  Gain=1/Ld
  Gain3 : Gain  Gain=-1/Ld
  Gain4 : Gain  Gain=LBG_K2
  Gain5 : Gain  Gain=-R/Ld
  Gain6 : Gain  Gain=LBG_K1
  Gain7 : Gain  Gain=1/Ld
  Gain8 : Gain  Gain=-1/Ld
  Gain9 : Gain  Gain=LBG_K2
  Product : Product
  Product1 : Product
  Sum : Sum  Inputs=++++
  Sum1 : Sum  Inputs=+-|
  Sum2 : Sum  Inputs=++++
  Sum3 : Sum  Inputs=+-|
  Unit Delay{,1..3} (4 alike) : UnitDelay  Commented=on  SampleTime=-1  HasFrameUpgradeWarning=on
  e_alpha_hat : Outport
  e_alpha_hat1 : Outport  Port=2
  wires:
  Sum/1 -> Discrete-Time Integrator7/1
  Gain/1 -> Sum/1
  Discrete-Time Integrator/1 -> Unit Delay/1
  Ialpha/1 -> Sum1/2
  Sum1/1 -> Gain1/1, Gain4/1
  Gain1/1 -> Sum/2
  [e_alpha_hat] -> Gain3/1
  ualpha/1 -> Gain2/1
  Gain2/1 -> Sum/3
  Gain3/1 -> Sum/4
  Add/1 -> Discrete-Time Integrator6/1
  we_lo/1 -> [we_lb]
  [we_lb] -> Product/1
  Discrete-Time Integrator2/1 -> Unit Delay2/1
  Product/1 -> Add/2
  Gain4/1 -> Add/1
  Discrete-Time Integrator1/1 -> Unit Delay1/1
  Sum2/1 -> Discrete-Time Integrator5/1
  Gain5/1 -> Sum2/1
  Gain6/1 -> Sum2/2
  Gain7/1 -> Sum2/3
  Gain8/1 -> Sum2/4
  Discrete-Time Integrator3/1 -> Unit Delay3/1
  Sum3/1 -> Gain6/1, Gain9/1
  Ibeta/1 -> Sum3/2
  Ubeta/1 -> Gain7/1
  [e_beta_hat] -> Gain8/1
  Add1/1 -> Discrete-Time Integrator4/1
  [we_lb] -> Product1/2
  Product1/1 -> Add1/1
  Gain9/1 -> Add1/2
  Discrete-Time Integrator4/1 -> [e_beta_hat], e_alpha_hat1/1, Product/2
  Discrete-Time Integrator5/1 -> Gain5/1, Sum3/1
  Discrete-Time Integrator6/1 -> e_alpha_hat/1, [e_alpha_hat], Product1/1
  Discrete-Time Integrator7/1 -> Gain/1, Sum1/1

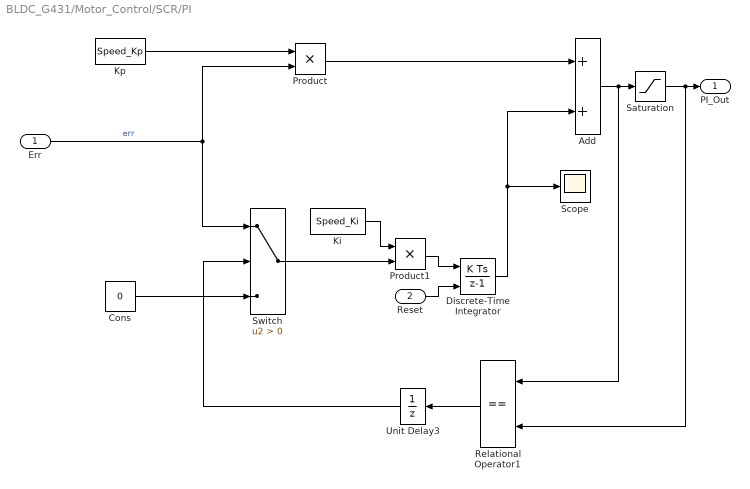
== system BLDC_G431/Motor_Control/SCR/PI ==
  Err : Inport
  Reset : Inport  Port=2
  Add : Sum
  Cons : Constant  Value=0  OutDataTypeStr=single
  Discrete-Time Integrator : DiscreteIntegrator  ExternalReset=level  SampleTime=-1  ICPrevOutput=DiscIntNeverNeededParam  ICPrevScaledInput=DiscIntNeverNeededParam
  Ki : Constant  Value=Speed_Ki  OutDataTypeStr=single
  Kp : Constant  Value=Speed_Kp  OutDataTypeStr=single
  Product : Product
  Product1 : Product
  Relational Operator1 : RelationalOperator  Operator===  OutDataTypeStr=boolean  RndMeth=Simplest
  Saturation : Saturate  UpperLimit=Speed_PI_OutputMax  LowerLimit=Speed_PI_OutputMin
  Scope : Scope
  Switch : Switch  Criteria=u2 > Threshold
  Unit Delay3 : UnitDelay  SampleTime=-1  HasFrameUpgradeWarning=on
  PI_Out : Outport
  wires:
  Kp/1 -> Product/1
  Err/1 -> Product/2, Switch/1  "err"
  Switch/1 -> Product1/2
  Product1/1 -> Discrete-Time Integrator/1
  Product/1 -> Add/1
  Add/1 -> Relational Operator1/1, Saturation/1
  Saturation/1 -> Relational Operator1/2, PI_Out/1
  Discrete-Time Integrator/1 -> Add/2, Scope/1
  Relational Operator1/1 -> Unit Delay3/1
  Ki/1 -> Product1/1
  Unit Delay3/1 -> Switch/2
  Cons/1 -> Switch/3
  Reset/1 -> Discrete-Time Integrator/2

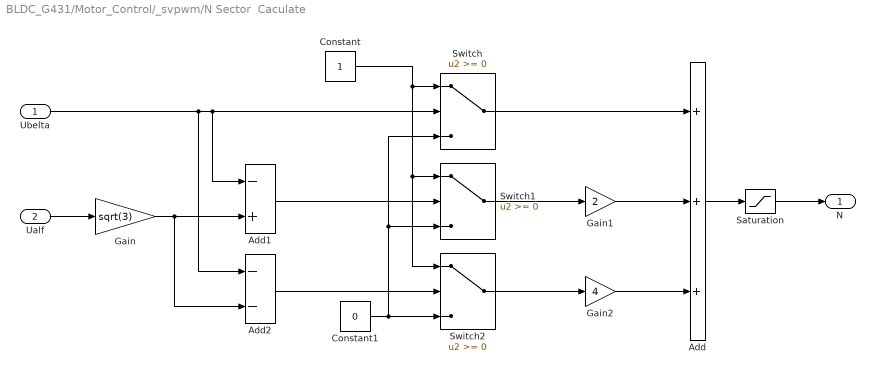
== system BLDC_G431/Motor_Control/_svpwm/N Sector  Caculate ==
  Ubelta : Inport
  Ualf : Inport  Port=2
  Add : Sum  Inputs=+++
  Add1 : Sum  Inputs=-+  OutDataTypeStr=single
  Add2 : Sum  Inputs=--  OutDataTypeStr=single
  Constant : Constant  OutDataTypeStr=single
  Constant1 : Constant  Value=0  OutDataTypeStr=single
  Gain : Gain  Gain=sqrt(3)
  Gain1 : Gain  Gain=2
  Gain2 : Gain  Gain=4
  Saturation : Saturate  UpperLimit=6  LowerLimit=1
  Switch : Switch
  Switch1 : Switch
  Switch2 : Switch
  N : Outport
  wires:
  Saturation/1 -> N/1
  Add/1 -> Saturation/1
  Gain2/1 -> Add/3
  Switch2/1 -> Gain2/1
  Add2/1 -> Switch2/2
  Gain1/1 -> Add/2
  Switch1/1 -> Gain1/1
  Add1/1 -> Switch1/2
  Gain/1 -> Add2/2, Add1/2
  Ualf/1 -> Gain/1
  Switch/1 -> Add/1
  Constant1/1 -> Switch/3, Switch1/3, Switch2/3
  Constant/1 -> Switch/1, Switch1/1, Switch2/1
  Ubelta/1 -> Add2/1, Add1/1, Switch/2

== system BLDC_G431/Motor_Control/_svpwm/Subsystem ==
  Ta : Inport
  Add : Sum  Inputs=+-
  Constant : Constant  Value=Tpwm  OutDataTypeStr=single
  Gain1 : Gain  Gain=2
  Gain4 : Gain  Gain=fpwm
  Da : Outport  OutDataTypeStr=single
  wires:
  Add/1 -> Gain4/1
  Gain1/1 -> Add/2
  Ta/1 -> Gain1/1
  Gain4/1 -> Da/1
  Constant/1 -> Add/1

== system BLDC_G431/Motor_Control/_svpwm/Subsystem1 ==
  Tb : Inport
  Add : Sum  Inputs=+-
  Constant : Constant  Value=Tpwm  OutDataTypeStr=single
  Gain1 : Gain  Gain=2
  Gain4 : Gain  Gain=fpwm
  Db : Outport  OutDataTypeStr=single
  wires:
  Constant/1 -> Add/1
  Gain4/1 -> Db/1
  Tb/1 -> Gain1/1
  Gain1/1 -> Add/2
  Add/1 -> Gain4/1

== system BLDC_G431/Motor_Control/_svpwm/Subsystem2 ==
  Tc : Inport
  Add : Sum  Inputs=+-
  Constant : Constant  Value=Tpwm  OutDataTypeStr=single
  Gain1 : Gain  Gain=2
  Gain4 : Gain  Gain=fpwm
  Dc : Outport  OutDataTypeStr=single
  wires:
  Add/1 -> Gain4/1
  Gain1/1 -> Add/2
  Tc/1 -> Gain1/1
  Gain4/1 -> Dc/1
  Constant/1 -> Add/1

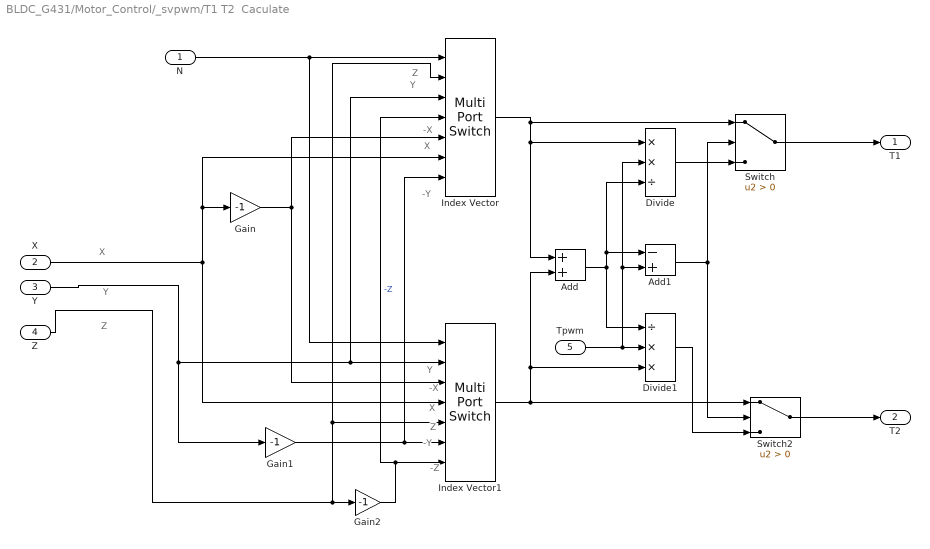
== system BLDC_G431/Motor_Control/_svpwm/T1 T2  Caculate ==
  note: Z
  note: Y
  note: -X
  note: X
  note: -Y
  note: Y
  note: -X
  note: X
  note: Z
  note: -Y
  note: -Z
  note: X
  note: Y
  note: Z
  N : Inport
  X : Inport  Port=2
  Y : Inport  Port=3
  Z : Inport  Port=4
  Tpwm : Inport  Port=5
  Add : Sum
  Add1 : Sum  Inputs=-+
  Divide : Product  Inputs=**/
  Divide1 : Product  Inputs=/**
  Gain : Gain  Gain=-1
  Gain1 : Gain  Gain=-1
  Gain2 : Gain  Gain=-1
  Index Vector : MultiPortSwitch  Inputs=6
  Index Vector1 : MultiPortSwitch  Inputs=6
  Switch : Switch  Criteria=u2 > Threshold
  Switch2 : Switch  Criteria=u2 > Threshold
  T1 : Outport
  T2 : Outport  Port=2
  wires:
  Switch2/1 -> T2/1
  Divide1/1 -> Switch2/3
  Switch/1 -> T1/1
  Add1/1 -> Switch/2, Switch2/2
  Add/1 -> Divide1/1, Divide/3, Add1/1
  Tpwm/1 -> Divide1/2, Divide/2, Add1/2
  Divide/1 -> Switch/3
  Index Vector1/1 -> Switch2/1, Add/2, Divide1/3
  Index Vector/1 -> Switch/1, Divide/1, Add/1
  Gain1/1 -> Index Vector/7, Index Vector1/6
  Gain2/1 -> Index Vector/4, Index Vector1/7  "-Z"
  Gain/1 -> Index Vector/5, Index Vector1/3
  Y/1 -> Gain1/1, Index Vector/3, Index Vector1/2
  X/1 -> Index Vector1/4, Index Vector/6, Gain/1
  Z/1 -> Index Vector/2, Index Vector1/5, Gain2/1
  N/1 -> Index Vector1/1, Index Vector/1

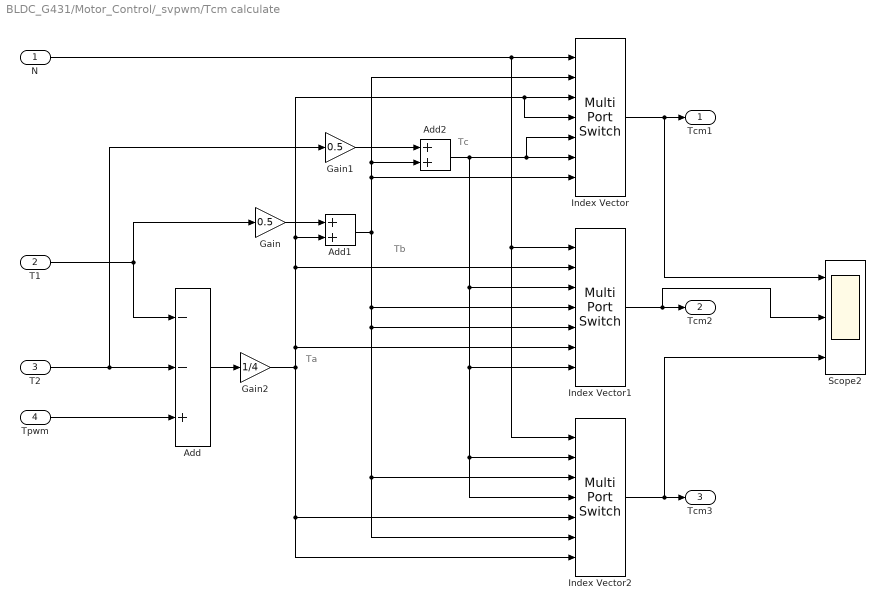
== system BLDC_G431/Motor_Control/_svpwm/Tcm calculate ==
  note: Tc
  note: Tb
  note: Ta
  N : Inport
  T1 : Inport  Port=2
  T2 : Inport  Port=3
  Tpwm : Inport  Port=4
  Add : Sum  Inputs=--+
  Add1 : Sum
  Add2 : Sum
  Gain : Gain  Gain=0.5
  Gain1 : Gain  Gain=0.5
  Gain2 : Gain  Gain=1/4
  Index Vector : MultiPortSwitch  Inputs=6
  Index Vector1 : MultiPortSwitch  Inputs=6
  Index Vector2 : MultiPortSwitch  Inputs=6
  Scope2 : Scope  NumInputPorts=3
  Tcm1 : Outport
  Tcm2 : Outport  Port=2
  Tcm3 : Outport  Port=3
  wires:
  Index Vector2/1 -> Scope2/3, Tcm3/1
  N/1 -> Index Vector/1, Index Vector1/1, Index Vector2/1
  Add2/1 -> Index Vector/5, Index Vector/6, Index Vector1/3, Index Vector1/7, Index Vector2/2, Index Vector2/4
  Gain1/1 -> Add2/1
  Add1/1 -> Add2/2, Index Vector/2, Index Vector/7, Index Vector1/4, Index Vector1/5, Index Vector2/3, Index Vector2/6
  Gain2/1 -> Index Vector2/5, Index Vector2/7, Add1/2, Index Vector/3, Index Vector/4, Index Vector1/2, Index Vector1/6
  Gain/1 -> Add1/1
  Add/1 -> Gain2/1
  Tpwm/1 -> Add/3
  T2/1 -> Add/2, Gain1/1
  T1/1 -> Add/1, Gain/1
  Index Vector/1 -> Scope2/1, Tcm1/1
  Index Vector1/1 -> Scope2/2, Tcm2/1

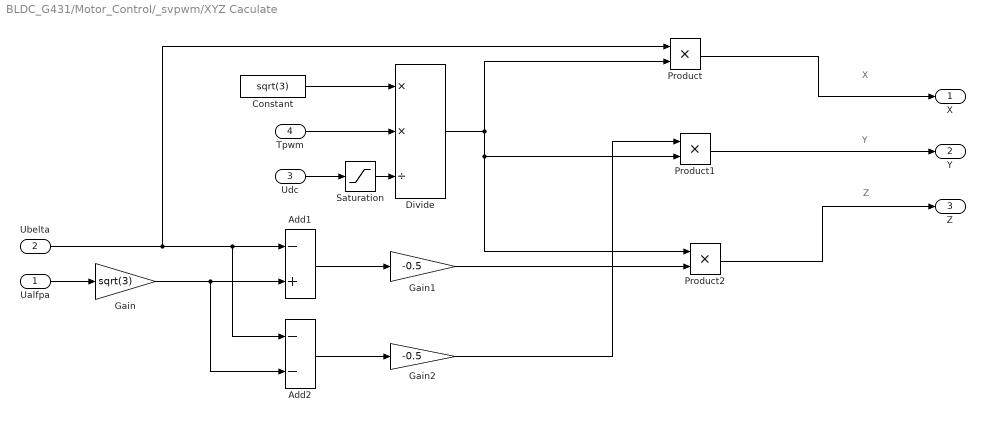
== system BLDC_G431/Motor_Control/_svpwm/XYZ Caculate ==
  note: X
  note: Y
  note: Z
  Ualfpa : Inport
  Ubelta : Inport  Port=2
  Udc : Inport  Port=3
  Tpwm : Inport  Port=4
  Add1 : Sum  Inputs=-+
  Add2 : Sum  Inputs=--
  Constant : Constant  Value=sqrt(3)  OutDataTypeStr=single
  Divide : Product  Inputs=**/
  Gain : Gain  Gain=sqrt(3)
  Gain1 : Gain  Gain=-0.5
  Gain2 : Gain  Gain=-0.5
  Product : Product
  Product1 : Product
  Product2 : Product
  Saturation : Saturate  UpperLimit=1200  LowerLimit=0.0001
  X : Outport
  Y : Outport  Port=2
  Z : Outport  Port=3
  wires:
  Gain2/1 -> Product1/1
  Add2/1 -> Gain2/1
  Add1/1 -> Gain1/1
  Gain/1 -> Add2/2, Add1/2
  Ualfpa/1 -> Gain/1
  Ubelta/1 -> Add2/1, Add1/1, Product/1
  Gain1/1 -> Product2/2
  Product2/1 -> Z/1
  Divide/1 -> Product1/2, Product2/1, Product/2
  Product1/1 -> Y/1
  Product/1 -> X/1
  Udc/1 -> Saturation/1
  Tpwm/1 -> Divide/2
  Constant/1 -> Divide/1
  Saturation/1 -> Divide/3

== system BLDC_G431/Motor_Control/Chart/close_loop/SCR/PI ==
  Err : Inport
  Reset : Inport  Port=2
  Add : Sum
  Cons : Constant  Value=0  OutDataTypeStr=single
  Discrete-Time Integrator : DiscreteIntegrator  ExternalReset=level  SampleTime=-1  ICPrevOutput=DiscIntNeverNeededParam  ICPrevScaledInput=DiscIntNeverNeededParam
  Ki : Constant  Value=Speed_Ki  OutDataTypeStr=single
  Kp : Constant  Value=Speed_Kp  OutDataTypeStr=single
  Product : Product
  Product1 : Product
  Relational Operator1 : RelationalOperator  Operator===  OutDataTypeStr=boolean  RndMeth=Simplest
  Saturation : Saturate  UpperLimit=Speed_PI_OutputMax  LowerLimit=Speed_PI_OutputMin
  Scope : Scope
  Switch : Switch  Criteria=u2 > Threshold
  Unit Delay3 : UnitDelay  SampleTime=-1  HasFrameUpgradeWarning=on
  PI_Out : Outport
  wires:
  Kp/1 -> Product/1
  Err/1 -> Product/2, Switch/1  "err"
  Switch/1 -> Product1/2
  Product1/1 -> Discrete-Time Integrator/1
  Product/1 -> Add/1
  Add/1 -> Relational Operator1/1, Saturation/1
  Saturation/1 -> Relational Operator1/2, PI_Out/1
  Discrete-Time Integrator/1 -> Add/2, Scope/1
  Relational Operator1/1 -> Unit Delay3/1
  Ki/1 -> Product1/1
  Unit Delay3/1 -> Switch/2
  Cons/1 -> Switch/3
  Reset/1 -> Discrete-Time Integrator/2

== system BLDC_G431/Motor_Control/Luenberger/PLL/Sine_Cosine ==
  note: Sine Cosine Coefficients
  P : Inport
  Cosine : Lookup_n-D  NumberOfTableDimensions=1  LookupTableObject=''  BreakpointsForDimension1=[0:2*pi/4095:2*pi]  BreakpointsForDimension1FirstPoint=10  BreakpointsForDimension2FirstPoint=10  BreakpointsForDimension1Spacing=12  BreakpointsForDimension2Spacing=12  IndexSearchMethod=Evenly spaced points  Table=Cosine_table  InterpMethod=Flat  DiagnosticForOutOfRangeInput=Error  InternalRulePriority=Speed  RndMeth=Simplest  InputSameDT=on
  Saturation : Saturate  UpperLimit=2*pi  LowerLimit=0
  Scope : Scope  NumInputPorts=2
  Sine : Lookup_n-D  NumberOfTableDimensions=1  LookupTableObject=''  BreakpointsForDimension1=[0:2*pi/4095:2*pi]  BreakpointsForDimension1FirstPoint=10  BreakpointsForDimension2FirstPoint=10  BreakpointsForDimension1Spacing=12  BreakpointsForDimension2Spacing=12  IndexSearchMethod=Evenly spaced points  Table=Sine_table  InterpMethod=Flat  DiagnosticForOutOfRangeInput=Error  InternalRulePriority=Speed  RndMeth=Simplest  InputSameDT=on
  Cos : Outport  VectorParamsAs1DForOutWhenUnconnected=off
  Sin : Outport  Port=2  VectorParamsAs1DForOutWhenUnconnected=off
  wires:
  P/1 -> Saturation/1  "position"
  Sine/1 -> Scope/1, Sin/1
  Cosine/1 -> Scope/2, Cos/1
  Saturation/1 -> Cosine/1, Sine/1

== system BLDC_G431/Motor_Control/Luenberger/PLL/SpeedToTheta ==
  In1 : Inport
  Angle_Limit : Subsystem
  Sum1 : Sum  Inputs=|++
  Ts : Gain  Gain=1/fpwm
  Unit Delay : UnitDelay  SampleTime=-1  HasFrameUpgradeWarning=on
  Theta : Outport
  wires:
  In1/1 -> Ts/1
  Ts/1 -> Sum1/1
  Sum1/1 -> Angle_Limit/1(Angle_input)
  Unit Delay/1 -> Theta/1, Sum1/2
  Angle_Limit/1(Angle_output) -> Unit Delay/1

== system BLDC_G431/Motor_Control/Luenberger/PLL/Subsystem1 ==
  Err_in : Inport
  speed : Inport  Port=2
  If : If
  If Action Subsystem : Subsystem  TreatAsAtomicUnit=on
  If Action Subsystem1 : Subsystem  TreatAsAtomicUnit=on
  Merge : Merge
  Product : Product
  Out : Outport  VectorParamsAs1DForOutWhenUnconnected=off
  wires:
  speed/1 -> If/1
  Merge/1 -> Product/1
  Err_in/1 -> Product/2
  Product/1 -> Out/1
  If/1 -> If Action Subsystem/Action
  If Action Subsystem/1(Out1) -> Merge/1
  If Action Subsystem1/1(Out1) -> Merge/2
  If/2 -> If Action Subsystem1/Action

== system BLDC_G431/Motor_Control/Luenberger/PLL/SpeedToTheta/Angle_Limit ==
  Angle_input : Inport
  If Action Subsystem1 : Subsystem  TreatAsAtomicUnit=on
  If Action Subsystem2 : Subsystem  TreatAsAtomicUnit=on
  If Action Subsystem3 : Subsystem  TreatAsAtomicUnit=on
  If1 : If  IfExpression=u1 > 6.283185307  ElseIfExpressions=u1<0
  Merge1 : Merge  Inputs=3
  Angle_output : Outport
  wires:
  If1/2 -> If Action Subsystem3/Action
  If1/1 -> If Action Subsystem2/Action
  If1/3 -> If Action Subsystem1/Action
  Merge1/1 -> Angle_output/1
  If Action Subsystem1/1(Out1) -> Merge1/3
  If Action Subsystem2/1(Out1) -> Merge1/1
  Angle_input/1 -> If Action Subsystem1/1(In1), If Action Subsystem2/1(In1), If Action Subsystem3/1(In1), If1/1
  If Action Subsystem3/1(Out1) -> Merge1/2

== system BLDC_G431/Motor_Control/Luenberger/PLL/Subsystem1/If Action Subsystem ==
  Action Port : ActionPort  ActionPortLabel=if(u1 > 0)
  Constant : Constant  OutDataTypeStr=single
  Out1 : Outport
  wires:
  Constant/1 -> Out1/1

== system BLDC_G431/Motor_Control/Luenberger/PLL/Subsystem1/If Action Subsystem1 ==
  Action Port : ActionPort  ActionPortLabel=else
  Constant : Constant  Value=-1  OutDataTypeStr=single
  Out1 : Outport
  wires:
  Constant/1 -> Out1/1

== system BLDC_G431/Motor_Control/Luenberger/PLL/SpeedToTheta/Angle_Limit/If Action Subsystem1 ==
  In1 : Inport
  Action Port : ActionPort  ActionPortLabel=else
  Out1 : Outport
  wires:
  In1/1 -> Out1/1

== system BLDC_G431/Motor_Control/Luenberger/PLL/SpeedToTheta/Angle_Limit/If Action Subsystem2 ==
  In1 : Inport
  Action Port : ActionPort  ActionPortLabel=if(u1 > 6.283185307)
  2pi : Constant  Value=2*pi  OutDataTypeStr=single
  Subtract1 : Sum  Inputs=+-  OutDataTypeStr=single
  Out1 : Outport
  wires:
  In1/1 -> Subtract1/1
  Subtract1/1 -> Out1/1
  2pi/1 -> Subtract1/2

== system BLDC_G431/Motor_Control/Luenberger/PLL/SpeedToTheta/Angle_Limit/If Action Subsystem3 ==
  In1 : Inport
  Action Port : ActionPort  ActionPortLabel=elseif(u1<0)
  Angle_offset : Constant  Value=2*pi  OutDataTypeStr=single
  Subtract1 : Sum
  Out1 : Outport
  wires:
  In1/1 -> Subtract1/1
  Subtract1/1 -> Out1/1
  Angle_offset/1 -> Subtract1/2

== stateflow chart BLDC_G431/Motor_Control/Chart ==
  state OPL
    [theta_fd1,iq_ref1] = open_loop(opl_spd,opl_time,opl_tor);
  state CLP
    [theta_fd1,iq_ref1] = close_loop(obs_spd,obs_theta,speed_ref);
  state AligStage
    theta_fd1 = 0;
    iq_ref1 = 1;
  state [theta_fd1,iq_ref1] = open_loop(opl_spd,opl_time,opl_tor) [function]
  state [theta_fd1,iq_ref1] = close_loop(obs_spd,obs_theta,speed_ref) [function]
  OPL -> CLP : [after(opl_time,sec) & obs_spd>800]
  AligStage -> OPL : [after(0.05,sec)]
  (default) -> AligStage
  data: opl_spd function_input single size=1; theta_fd1 function_output single; iq_ref1 function_output single; opl_time function_input single size=1; opl_tor function_input single size=1; obs_spd function_input single size=1; obs_theta function_input single size=1; speed_ref function_input single size=1; theta_fd1 function_output single; iq_ref1 function_output single; obs_spd input single; speed_ref input single; obs_theta input single; iq_ref1 output single; theta_fd1 output single; opl_time input single; opl_spd input single; opl_tor input single
  events: event input FUNCTION_CALL_EVENT
